simulink model "per3"  (R2019b)
settings: Solver=FixedStepAuto  StartTime=0.0  StopTime=inf  RelTol=1e-3  EnableMultiTasking=on
libraries: instrumentlib x1
settings Model: SILPILModeSetting=veronly  ExtModeTrigDuration=2  Creator=user  LastModifiedBy=user
settings OptimizationCC: EnhancedBackFolding=on  PassReuseOutputArgsAs=Individual arguments  ZeroExternalMemoryAtStartup=off  ZeroInternalMemoryAtStartup=off  MaxStackSize=64  OptimizeBlockOrder=speed  DifferentSizesBufferReuse=on  OptimizationCustomize=off  EfficientTunableParamExpr=on
settings DebuggingCC: ParameterTunabilityLossMsg=error
settings HardwareCC: ProdBitPerInt=16  ProdBitPerPointer=16  ProdBitPerSizeT=16  ProdBitPerPtrDiffT=16  ProdLargestAtomicFloat=None  ProdWordSize=8  ProdHWDeviceType=Atmel->AVR
settings SFSimCC: MATLABDynamicMemAlloc=off
settings RTWCC: SystemTargetFile=ert.tlc  HardwareBoard=Arduino Mega 2560  TLCOptions=-aInlineSetEventsForThisBaseRateFcn=TLC_FALSE -aSuppressMultiTaskScheduler=TLC_FALSE -aRateBasedStepFcn=1  TemplateMakefile=ert_default_tmf  GenerateReport=on  Toolchain=Arduino AVR  BuildConfiguration=Faster Runs  IncludeHyperlinkInReport=on  LaunchReport=on  GenerateTraceInfo=on  GenerateTraceReport=on  GenerateTraceReportSl=on  GenerateTraceReportSf=on  GenerateTraceReportEml=on
settings CodeAppCC: ForceParamTrailComments=on  IgnoreCustomStorageClasses=off  OperatorAnnotations=on  SimulinkDataObjDesc=on  SFDataObjDesc=on  InsertBlockDesc=on
settings ERTTargetCC: DynamicStringBufferSize=512  SupportContinuousTime=on  SupportVariableSizeSignals=on  ExtModeStaticAllocSize=2048

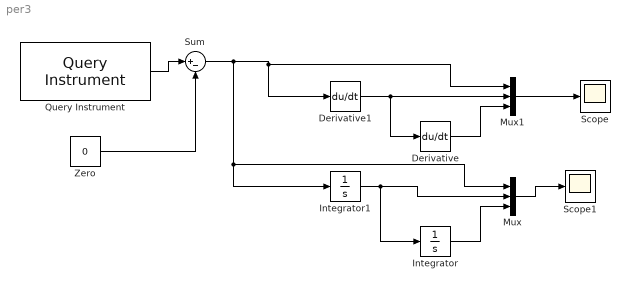
== system per3 ==
  Derivative : Derivative
  Derivative1 : Derivative
  Integrator : Integrator
  Integrator1 : Integrator
  Mux : Mux  Inputs=3
  Mux1 : Mux  Inputs=3
  Query Instrument : instrumentlib/Query Instrument  sampleTime=1  isWorkspaceObject=off  timeout=10  inputBufferSize=512  protocol=Serial  serialPort=COM4  baudRate=9600  gpibVendor=Keysight Technologies  boardIndex=0  primaryAddress=1  secondaryAddress=0  visaVendor=Keysight  visaSerialPort=0  chassisIndex=0  logicalAddress=0  tcpRemoteHost='127.0.0.1'  tcpRemotePort=4500  udpRemoteHost='127.0.0.1'  udpRemotePort=9090  visaTCPBoardIndex=0  visaTCPRemoteHost='127.0.0.1'  usbBoardIndex=0  usbManufID=0  usbModelCode=0  usbSerialNumber=0  initAction=None  initCommand='DATA:SOURCE CH1'  initFunction=get  queryCommand='curve?'  responseFormat=ASCII  asciiFormatting='%d,'  precision=8-bit integer  byteOrder=Little endian  valuesToRead=1  removeBytes=off  afterOutputAction=Repeat query for new data  enableFrames=off  frameSize=1
      settings: SourceProductName=Instrument Control Toolbox  SourceProductBaseCode=IC
  Scope : Scope
  Scope1 : Scope
  Sum : Sum  Inputs=|+-
  Zero : Constant  Value=0  OutDataTypeStr=Inherit: Inherit via back propagation
  wires:
  Zero/1 -> Sum/2
  Sum/1 -> Mux/1, Integrator1/1, Mux1/1, Derivative1/1
  Derivative1/1 -> Mux1/2, Derivative/1
  Derivative/1 -> Mux1/3
  Mux1/1 -> Scope/1
  Mux/1 -> Scope1/1
  Integrator1/1 -> Integrator/1, Mux/2
  Integrator/1 -> Mux/3
  Query Instrument/1 -> Sum/1
